simulink model "run_sim_paper_scenario"  (R2020a)
settings: Solver=ode4  StartTime=0.0  StopTime=30.0  FixedStep=0.01  RelTol=1e-3
values from neighbouring files (symbols this model uses):
  alfa_theta = 20    [init_sim_paper_scenario.m]
  alfa_theta_obs = 100    [init_sim_paper_scenario.m]
  beta1 = 1.2    [init_sim_paper_scenario.m]
  beta2 = 0.8    [init_sim_paper_scenario.m]
  beta_Phi_1 = pp0 * cal_frac_squ( 3, p_p0_plus_1, q_p0_plus_1 )                          * cal_frac_squ( eps_s_bar / pi, p_p0_min_2, q_p0_min_2 )                          / ( 2 * ( 2 * pp0 - 1 ) * tanh( gamma0 * ( eps_s_bar / pi ) / 2 ) )                          - ( cal_frac_squ( 3, p_p0_plus_1, q_p0_plus_1 ) * gamma0 / ( 4 * ( 2 * pp0 -1 ) ) )                          * cal_frac_squ( eps_s_bar / pi, p_p0_min_ ...(+136 chars)    [init_sim_paper_scenario.m]
  beta_Phi_2 = ( 1 - pp0 ) * cal_frac_squ( 3, p_p0_plus_1, q_p0_plus_1 )                          / ( 2 * ( 1 - 2 * pp0 ) * cal_frac_squ( eps_s_bar / pi, p_p0_0, q_p0_0 ) * tanh( gamma0 * ( eps_s_bar / pi ) / 2 ) )                          - ( cal_frac_squ( 3, p_p0_plus_1, q_p0_plus_1 ) * gamma0 / ( 4 * ( 1 - 2 * pp0 ) ) )                          * cal_frac_squ( eps_s_bar / pi, p_1_min_p0, q_1_min_p0 )          ...(+112 chars)    [init_sim_paper_scenario.m]
  c1_diff_sigma_bar_v = diag([25; 30; 20])    [init_sim_paper_scenario.m]
  c1_diff_sigma_bar_w = diag([12; 12; 12])    [init_sim_paper_scenario.m]
  c1_diff_ui = diag([25; 30; 20])    [init_sim_paper_scenario.m]
  c1v = diag([5.8; 6.5; 6.5])    [init_sim_paper_scenario.m]
  c2_diff_sigma_bar_v = diag([50; 50; 10])    [init_sim_paper_scenario.m]
  c2_diff_sigma_bar_w = diag([12; 12; 12])    [init_sim_paper_scenario.m]
  c2_diff_ui = diag([50; 50; 10])    [init_sim_paper_scenario.m]
  c2v = diag([5.8; 6.5; 6.5])    [init_sim_paper_scenario.m]
  c3_diff_sigma_bar_v = diag([15; 15; 10])    [init_sim_paper_scenario.m]
  c3_diff_sigma_bar_w = diag([15; 15; 15])    [init_sim_paper_scenario.m]
  c3_diff_ui = diag([15; 15; 10])    [init_sim_paper_scenario.m]
  c3v = diag([4.8; 6.4; 6.0])    [init_sim_paper_scenario.m]
  c_w_1 = diag( [20; 15; 15] )    [init_sim_paper_scenario.m]
  c_w_2 = diag( [20; 15; 15] )    [init_sim_paper_scenario.m]
  c_w_3 = diag( [2; 2; 2] )    [init_sim_paper_scenario.m]
  cS0 = diag( [4.5; 4.5; 4.5] )    [init_sim_paper_scenario.m]
  delta_p_i_0 = zeros(3, NF)    [init_sim_paper_scenario.m]
  delta_v_i_0 = zeros(3, NF)    [init_sim_paper_scenario.m]
  dp_aa_t = 0.2 * ones(3, 5) + ( 1.0 - 0.2 ) * rand(3, 5)    [init_sim_paper_scenario.m]
  dp_ff_t = [ 0.4 * ones(1, 5) + ( 1.0 - 0.4 ) * rand(1, 5);                      0.4 * ones(1, 5) + ( 1.0 - 0.4 ) * rand(1, 5);                      0.2 * ones(1, 5) + ( 0.6 - 0.2 ) * rand(1, 5) ]    [init_sim_paper_scenario.m]
  dp_phi_t = ( - pi / 2 ) * ones(3, 5) + ( pi / 2 - ( - pi / 2 ) ) * rand(3, 5)    [init_sim_paper_scenario.m]
  dw_aa_t = 0.2 * ones(3, 5) + ( 1.0 - 0.2 ) * rand(3, 5)    [init_sim_paper_scenario.m]
  dw_ff_t = [ 0.4 * ones(1, 5) + ( 1.0 - 0.4 ) * rand(1, 5);                      0.4 * ones(1, 5) + ( 1.0 - 0.4 ) * rand(1, 5);                      0.2 * ones(1, 5) + ( 0.6 - 0.2 ) * rand(1, 5) ]    [init_sim_paper_scenario.m]
  dw_phi_t = ( - pi / 2 ) * ones(3, 5) + ( pi / 2 - ( - pi / 2 ) ) * rand(3, 5)    [init_sim_paper_scenario.m]
  dwci_init = zeros(3,5)    [init_sim_paper_scenario.m]
  eps_s_bar_div_pi = eps_s_bar / pi    (= 0.03)    [init_sim_paper_scenario.m]
  etai_0 = zeros(3,5)    [init_sim_paper_scenario.m]
  gamma0 = 20    [init_sim_paper_scenario.m]
  h1w = diag([20.0; 20.0; 20.0])    [init_sim_paper_scenario.m]
  h2w = diag([30.0; 35.0; 35.0])    [init_sim_paper_scenario.m]
  h3w = diag([30.0; 25.0; 30.0])    [init_sim_paper_scenario.m]
  Ji = zeros(3,3,NF)    [init_sim_paper_scenario.m]
  k_J_0 = diag( [1; 1; 1] )    [init_sim_paper_scenario.m]
  kai_1_t = 0.02    [init_sim_paper_scenario.m]
  kai_3_t = 0.1    [init_sim_paper_scenario.m]
  kai_chi_1 = diag([6; 6; 6])    [init_sim_paper_scenario.m]
  kai_chi_2 = diag([6; 6; 6])    [init_sim_paper_scenario.m]
  kai_u_1 = diag([8; 8; 8])    [init_sim_paper_scenario.m]
  kai_u_2 = diag([8; 8; 8])    [init_sim_paper_scenario.m]
  ksii_0 = zeros(3,5)    [init_sim_paper_scenario.m]
  l1v = diag([20; 20; 20])    [init_sim_paper_scenario.m]
  l2v = diag([30; 30; 30])    [init_sim_paper_scenario.m]
  Lamd_diff_sigma_bar_v = 0.5    [init_sim_paper_scenario.m]
  Lamd_diff_sigma_bar_w = 0.8    [init_sim_paper_scenario.m]
  Lamd_diff_ui = 0.8    [init_sim_paper_scenario.m]
  mass_i = zeros(1,NF)    [init_sim_paper_scenario.m]
  Mii = diag([1;0;0;0;1])    [init_sim_paper_scenario.m]
  mu_c_theta = 100    [init_sim_paper_scenario.m]
  mu_d_w = 100    [init_sim_paper_scenario.m]
  pos0 = zeros(3, 1)    [init_sim_paper_scenario.m]
  pp0 = 8 / 11    (= 0.727272727273)    [init_sim_paper_scenario.m]    (also in plot_sim_paper_scenario.m = plot3( ksi0(1, kkt), ksi0(2, kkt), ksi0(3, kkt),            )
  PZ0 = P0(3)    [init_sim_paper_scenario.m]
  PZ1 = 10    [init_sim_paper_scenario.m]
  Qci_init = repmat([1;0;0;0],1,NF)    [init_sim_paper_scenario.m]
  R0 = 4    [init_sim_paper_scenario.m]
  R1 = 8    [init_sim_paper_scenario.m]
  Rci_init = zeros(3,3,NF)    [init_sim_paper_scenario.m]
  Ri_init = zeros(3,3,NF)    [init_sim_paper_scenario.m]
  Rx2 = 10    [init_sim_paper_scenario.m]
  Ry2 = 6    [init_sim_paper_scenario.m]
  Rz2 = 4    [init_sim_paper_scenario.m]
  T0 = 0    [init_sim_paper_scenario.m]
  T1 = tseq1    (= 10)    [init_sim_paper_scenario.m]
  T12 = tseq1 + tseq12    (= 20)    [init_sim_paper_scenario.m]
  T2 = tseq1 + tseq12 + tseq2    (= 30)    [init_sim_paper_scenario.m]
  theta0 = ( 2 / 5 ) * pi    (= 1.25663706144)    [init_sim_paper_scenario.m]
  thr_p_plus_1 = cal_frac_squ( 3, p_p0_plus_1, q_p0_plus_1 )    [init_sim_paper_scenario.m]
  ui_init = zeros(3,NF)    [init_sim_paper_scenario.m]
  vel0 = zeros(3, 1)    [init_sim_paper_scenario.m]
  wci_init = zeros(3,5)    [init_sim_paper_scenario.m]
  Wij = [0,0,1,0,0;              0,0,1,1,0;              1,0,0,0,1;              0,1,1,0,0;              0,0,1,0,0]    [init_sim_paper_scenario.m]
  X1 = 8    [init_sim_paper_scenario.m]
  X2 = 2    [init_sim_paper_scenario.m]
  X3 = 3    [init_sim_paper_scenario.m]
  Y1 = 10    [init_sim_paper_scenario.m]
  Y2 = 2    [init_sim_paper_scenario.m]
  Y3 = 4    [init_sim_paper_scenario.m]
  Z1 = 4    [init_sim_paper_scenario.m]
  Z2 = -6    [init_sim_paper_scenario.m]
  Z3 = 2    [init_sim_paper_scenario.m]
  zeta_diff_sigma_bar_v = 0.08    [init_sim_paper_scenario.m]
  zeta_diff_sigma_bar_w = 0.3    [init_sim_paper_scenario.m]
  zeta_diff_ui = 0.05    [init_sim_paper_scenario.m]
undefined symbols (not defined in the file or in its folder): cal_frac_squ, p_2_p0, p_alfav1, p_alfav2, p_alfaw1, p_alfaw2, p_beta1, p_beta2, p_beta_w_1, p_beta_w_2, p_dbeta1, p_dbeta2, p_gamma1_pos, p_gamma1_vel, p_gamma2_pos, p_gamma2_vel, p_p0_min_1, p_p0_plus_1, q_2_p0, q_alfav1, q_alfav2, q_alfaw1, q_alfaw2, q_beta1, q_beta2, q_beta_w_1, q_beta_w_2, q_dbeta1, q_dbeta2, q_gamma1_pos, q_gamma1_vel, q_gamma2_pos, q_gamma2_vel, q_p0_min_1, q_p0_plus_1, Qei_init, Qi_init, Rei_init, V_Phi_Rei_init, wei_init, wi_init
(part 9 of 10)

== matlab function run_sim_paper_scenario/cal taui agent 1 ==
  data: c_w_1 input; c_w_2 input; c_w_3 input; k_J_0 input; tau_1 output; Ji input; Si_vec input; dw_hat_vec input; Fi_S_vec input; theta_Si_beta_w_1_vec input; theta_Si_beta_w_2_vec input
function tau_1 = fcn(c_w_1, c_w_2, c_w_3, k_J_0, Ji, Si_vec, dw_hat_vec, ...
                                        Fi_S_vec, theta_Si_beta_w_1_vec, theta_Si_beta_w_2_vec)
%%%% applied torque control input for rotational subsystem
iiuav = 1;
tau_1 = -c_w_1 * theta_Si_beta_w_1_vec(:,iiuav) - c_w_2 * theta_Si_beta_w_2_vec(:,iiuav) - c_w_3 * Si_vec(:,iiuav) ...
                - dw_hat_vec(:,iiuav) - k_J_0 * inv( Ji(:,:,iiuav) ) * Fi_S_vec(:,iiuav);
end

== matlab function run_sim_paper_scenario/cal taui agent 2 ==
  data: c_w_1 input; c_w_2 input; c_w_3 input; k_J_0 input; tau_2 output; Ji input; Si_vec input; dw_hat_vec input; Fi_S_vec input; theta_Si_beta_w_1_vec input; theta_Si_beta_w_2_vec input
function tau_2 = fcn(c_w_1, c_w_2, c_w_3, k_J_0, Ji, Si_vec, dw_hat_vec, ...
                                        Fi_S_vec, theta_Si_beta_w_1_vec, theta_Si_beta_w_2_vec)
%%%% applied torque control input for rotational subsystem
iiuav = 2;
tau_2 = -c_w_1 * theta_Si_beta_w_1_vec(:,iiuav) - c_w_2 * theta_Si_beta_w_2_vec(:,iiuav) - c_w_3 * Si_vec(:,iiuav) ...
                - dw_hat_vec(:,iiuav) - k_J_0 * inv( Ji(:,:,iiuav) ) * Fi_S_vec(:,iiuav);
end

== matlab function run_sim_paper_scenario/cal taui agent 3 ==
  data: c_w_1 input; c_w_2 input; c_w_3 input; k_J_0 input; tau_3 output; Ji input; Si_vec input; dw_hat_vec input; Fi_S_vec input; theta_Si_beta_w_1_vec input; theta_Si_beta_w_2_vec input
function tau_3 = fcn(c_w_1, c_w_2, c_w_3, k_J_0, Ji, Si_vec, dw_hat_vec, ...
                                        Fi_S_vec, theta_Si_beta_w_1_vec, theta_Si_beta_w_2_vec)
%%%% applied torque control input for rotational subsystem
iiuav = 3;
tau_3 = -c_w_1 * theta_Si_beta_w_1_vec(:,iiuav) - c_w_2 * theta_Si_beta_w_2_vec(:,iiuav) - c_w_3 * Si_vec(:,iiuav) ...
                - dw_hat_vec(:,iiuav) - k_J_0 * inv( Ji(:,:,iiuav) ) * Fi_S_vec(:,iiuav);
end

== matlab function run_sim_paper_scenario/cal taui agent 4 ==
  data: c_w_1 input; c_w_2 input; c_w_3 input; k_J_0 input; tau_4 output; Ji input; Si_vec input; dw_hat_vec input; Fi_S_vec input; theta_Si_beta_w_1_vec input; theta_Si_beta_w_2_vec input
function tau_4 = fcn(c_w_1, c_w_2, c_w_3, k_J_0, Ji, Si_vec, dw_hat_vec, ...
                                        Fi_S_vec, theta_Si_beta_w_1_vec, theta_Si_beta_w_2_vec)
%%%% applied torque control input for rotational subsystem
iiuav = 4;
tau_4 = -c_w_1 * theta_Si_beta_w_1_vec(:,iiuav) - c_w_2 * theta_Si_beta_w_2_vec(:,iiuav) - c_w_3 * Si_vec(:,iiuav) ...
                - dw_hat_vec(:,iiuav) - k_J_0 * inv( Ji(:,:,iiuav) ) * Fi_S_vec(:,iiuav);
end

== matlab function run_sim_paper_scenario/cal taui agent 5 ==
  data: c_w_1 input; c_w_2 input; c_w_3 input; k_J_0 input; tau_5 output; Ji input; Si_vec input; dw_hat_vec input; Fi_S_vec input; theta_Si_beta_w_1_vec input; theta_Si_beta_w_2_vec input
function tau_5 = fcn(c_w_1, c_w_2, c_w_3, k_J_0, Ji, Si_vec, dw_hat_vec, ...
                                        Fi_S_vec, theta_Si_beta_w_1_vec, theta_Si_beta_w_2_vec)
%%%% applied torque control input for rotational subsystem
iiuav = 5;
tau_5 = -c_w_1 * theta_Si_beta_w_1_vec(:,iiuav) - c_w_2 * theta_Si_beta_w_2_vec(:,iiuav) - c_w_3 * Si_vec(:,iiuav) ...
                - dw_hat_vec(:,iiuav) - k_J_0 * inv( Ji(:,:,iiuav) ) * Fi_S_vec(:,iiuav);
end

== matlab function run_sim_paper_scenario/cal theta_Si_beta_w agent 1 ==
  data: mu_c_theta input; Si_squ_beta_w_1_vec input; theta_Si_beta_w_1_node_1 output; Si_squ_beta_w_2_vec input; Si_vec input; theta_Si_beta_w_2_node_1 output
function [theta_Si_beta_w_1_node_1, theta_Si_beta_w_2_node_1] = fcn(mu_c_theta, Si_squ_beta_w_1_vec, Si_squ_beta_w_2_vec, Si_vec)
iiuav = 1;
theta_Si_beta_w_1_node_1 = Si_squ_beta_w_1_vec(:, iiuav) .* ( -1 + 2 ./ ( 1 + exp( -mu_c_theta .* Si_vec(:,iiuav) ) ) );
theta_Si_beta_w_2_node_1 = Si_squ_beta_w_2_vec(:, iiuav) .* ( -1 + 2 ./ ( 1 + exp( -mu_c_theta .* Si_vec(:,iiuav) ) ) );

== matlab function run_sim_paper_scenario/cal theta_Si_beta_w agent 2 ==
  data: mu_c_theta input; Si_squ_beta_w_1_vec input; theta_Si_beta_w_1_node_2 output; Si_squ_beta_w_2_vec input; Si_vec input; theta_Si_beta_w_2_node_2 output
function [theta_Si_beta_w_1_node_2, theta_Si_beta_w_2_node_2] = fcn(mu_c_theta, Si_squ_beta_w_1_vec, Si_squ_beta_w_2_vec, Si_vec)
iiuav = 2;
theta_Si_beta_w_1_node_2 = Si_squ_beta_w_1_vec(:, iiuav) .* ( -1 + 2 ./ ( 1 + exp( -mu_c_theta .* Si_vec(:,iiuav) ) ) );
theta_Si_beta_w_2_node_2 = Si_squ_beta_w_2_vec(:, iiuav) .* ( -1 + 2 ./ ( 1 + exp( -mu_c_theta .* Si_vec(:,iiuav) ) ) );

== matlab function run_sim_paper_scenario/combine follower eta ksi ==
  data: ksi_track_err_vec output; ksi_track_err_1 input; ksi_track_err_2 input; ksi_track_err_3 input; ksi_track_err_4 input; ksi_track_err_5 input; eta_track_err_vec output; eta_track_err_1 input; eta_track_err_2 input; eta_track_err_3 input; eta_track_err_4 input; eta_track_err_5 input
function [ksi_track_err_vec, eta_track_err_vec]  = fcn(ksi_track_err_1, ksi_track_err_2, ksi_track_err_3, ksi_track_err_4, ksi_track_err_5, ...
                                                                                    eta_track_err_1, eta_track_err_2, eta_track_err_3, eta_track_err_4, eta_track_err_5)
ksi_track_err_vec = [ksi_track_err_1(:), ksi_track_err_2(:), ksi_track_err_3(:), ksi_track_err_4(:), ksi_track_err_5(:)];
eta_track_err_vec = [eta_track_err_1(:), eta_track_err_2(:), eta_track_err_3(:), eta_track_err_4(:), eta_track_err_5(:)];

== matlab function run_sim_paper_scenario/cal theta_Si_beta_w agent 3 ==
  data: mu_c_theta input; Si_squ_beta_w_1_vec input; theta_Si_beta_w_1_node_3 output; Si_squ_beta_w_2_vec input; Si_vec input; theta_Si_beta_w_2_node_3 output
function [theta_Si_beta_w_1_node_3, theta_Si_beta_w_2_node_3] = fcn(mu_c_theta, Si_squ_beta_w_1_vec, Si_squ_beta_w_2_vec, Si_vec)
iiuav = 3;
theta_Si_beta_w_1_node_3 = Si_squ_beta_w_1_vec(:, iiuav) .* ( -1 + 2 ./ ( 1 + exp( -mu_c_theta .* Si_vec(:,iiuav) ) ) );
theta_Si_beta_w_2_node_3 = Si_squ_beta_w_2_vec(:, iiuav) .* ( -1 + 2 ./ ( 1 + exp( -mu_c_theta .* Si_vec(:,iiuav) ) ) );

== matlab function run_sim_paper_scenario/cal theta_Si_beta_w agent 4 ==
  data: mu_c_theta input; Si_squ_beta_w_1_vec input; theta_Si_beta_w_1_node_4 output; Si_squ_beta_w_2_vec input; Si_vec input; theta_Si_beta_w_2_node_4 output
function [theta_Si_beta_w_1_node_4, theta_Si_beta_w_2_node_4] = fcn(mu_c_theta, Si_squ_beta_w_1_vec, Si_squ_beta_w_2_vec, Si_vec)
iiuav = 4;
theta_Si_beta_w_1_node_4 = Si_squ_beta_w_1_vec(:, iiuav) .* ( -1 + 2 ./ ( 1 + exp( -mu_c_theta .* Si_vec(:,iiuav) ) ) );
theta_Si_beta_w_2_node_4 = Si_squ_beta_w_2_vec(:, iiuav) .* ( -1 + 2 ./ ( 1 + exp( -mu_c_theta .* Si_vec(:,iiuav) ) ) );

== matlab function run_sim_paper_scenario/cal theta_Si_beta_w agent 5 ==
  data: mu_c_theta input; Si_squ_beta_w_1_vec input; theta_Si_beta_w_1_node_5 output; Si_squ_beta_w_2_vec input; Si_vec input; theta_Si_beta_w_2_node_5 output
function [theta_Si_beta_w_1_node_5, theta_Si_beta_w_2_node_5] = fcn(mu_c_theta, Si_squ_beta_w_1_vec, Si_squ_beta_w_2_vec, Si_vec)
iiuav = 5;
theta_Si_beta_w_1_node_5 = Si_squ_beta_w_1_vec(:, iiuav) .* ( -1 + 2 ./ ( 1 + exp( -mu_c_theta .* Si_vec(:,iiuav) ) ) );
theta_Si_beta_w_2_node_5 = Si_squ_beta_w_2_vec(:, iiuav) .* ( -1 + 2 ./ ( 1 + exp( -mu_c_theta .* Si_vec(:,iiuav) ) ) );

== matlab function run_sim_paper_scenario/cal theta_sigma_bar_w_tilt agent 1 ==
  data: alfa_theta_obs_w input; sigma_bar_w_tilt_squ_1_1 input; theta_sigma_bar_w_tilt_1_1 output; sigma_bar_w_tilt_squ_2_1 input; sigma_bar_w_tilt_vec input; theta_sigma_bar_w_tilt_2_1 output
function [theta_sigma_bar_w_tilt_1_1, theta_sigma_bar_w_tilt_2_1] = fcn(alfa_theta_obs_w, sigma_bar_w_tilt_squ_1_1, sigma_bar_w_tilt_squ_2_1, sigma_bar_w_tilt_vec)
iiuav = 1;
theta_sigma_bar_w_tilt_1_1 = sigma_bar_w_tilt_squ_1_1(:) .* ( -1 + 2 ./ ( 1 + exp( -alfa_theta_obs_w .* sigma_bar_w_tilt_vec(:,iiuav) ) ) );
theta_sigma_bar_w_tilt_2_1 = sigma_bar_w_tilt_squ_2_1(:) .* ( -1 + 2 ./ ( 1 + exp( -alfa_theta_obs_w .* sigma_bar_w_tilt_vec(:,iiuav) ) ) );

== matlab function run_sim_paper_scenario/cal theta_sigma_bar_w_tilt agent 2 ==
  data: alfa_theta_obs_w input; sigma_bar_w_tilt_squ_1_2 input; theta_sigma_bar_w_tilt_1_2 output; sigma_bar_w_tilt_squ_2_2 input; sigma_bar_w_tilt_vec input; theta_sigma_bar_w_tilt_2_2 output
function [theta_sigma_bar_w_tilt_1_2, theta_sigma_bar_w_tilt_2_2] = fcn(alfa_theta_obs_w, sigma_bar_w_tilt_squ_1_2, sigma_bar_w_tilt_squ_2_2, sigma_bar_w_tilt_vec)
iiuav = 2;
theta_sigma_bar_w_tilt_1_2 = sigma_bar_w_tilt_squ_1_2(:) .* ( -1 + 2 ./ ( 1 + exp( -alfa_theta_obs_w .* sigma_bar_w_tilt_vec(:,iiuav) ) ) );
theta_sigma_bar_w_tilt_2_2 = sigma_bar_w_tilt_squ_2_2(:) .* ( -1 + 2 ./ ( 1 + exp( -alfa_theta_obs_w .* sigma_bar_w_tilt_vec(:,iiuav) ) ) );

== matlab function run_sim_paper_scenario/cal theta_sigma_bar_w_tilt agent 3 ==
  data: alfa_theta_obs_w input; sigma_bar_w_tilt_squ_1_3 input; theta_sigma_bar_w_tilt_1_3 output; sigma_bar_w_tilt_squ_2_3 input; sigma_bar_w_tilt_vec input; theta_sigma_bar_w_tilt_2_3 output
function [theta_sigma_bar_w_tilt_1_3, theta_sigma_bar_w_tilt_2_3] = fcn(alfa_theta_obs_w, sigma_bar_w_tilt_squ_1_3, sigma_bar_w_tilt_squ_2_3, sigma_bar_w_tilt_vec)
iiuav = 3;
theta_sigma_bar_w_tilt_1_3 = sigma_bar_w_tilt_squ_1_3(:) .* ( -1 + 2 ./ ( 1 + exp( -alfa_theta_obs_w .* sigma_bar_w_tilt_vec(:,iiuav) ) ) );
theta_sigma_bar_w_tilt_2_3 = sigma_bar_w_tilt_squ_2_3(:) .* ( -1 + 2 ./ ( 1 + exp( -alfa_theta_obs_w .* sigma_bar_w_tilt_vec(:,iiuav) ) ) );

== matlab function run_sim_paper_scenario/cal theta_sigma_bar_w_tilt agent 4 ==
  data: alfa_theta_obs_w input; sigma_bar_w_tilt_squ_1_4 input; theta_sigma_bar_w_tilt_1_4 output; sigma_bar_w_tilt_squ_2_4 input; sigma_bar_w_tilt_vec input; theta_sigma_bar_w_tilt_2_4 output
function [theta_sigma_bar_w_tilt_1_4, theta_sigma_bar_w_tilt_2_4] = fcn(alfa_theta_obs_w, sigma_bar_w_tilt_squ_1_4, sigma_bar_w_tilt_squ_2_4, sigma_bar_w_tilt_vec)
iiuav = 4;
theta_sigma_bar_w_tilt_1_4 = sigma_bar_w_tilt_squ_1_4(:) .* ( -1 + 2 ./ ( 1 + exp( -alfa_theta_obs_w .* sigma_bar_w_tilt_vec(:,iiuav) ) ) );
theta_sigma_bar_w_tilt_2_4 = sigma_bar_w_tilt_squ_2_4(:) .* ( -1 + 2 ./ ( 1 + exp( -alfa_theta_obs_w .* sigma_bar_w_tilt_vec(:,iiuav) ) ) );

== matlab function run_sim_paper_scenario/cal theta_sigma_bar_w_tilt agent 5 ==
  data: alfa_theta_obs_w input; sigma_bar_w_tilt_squ_1_5 input; theta_sigma_bar_w_tilt_1_5 output; sigma_bar_w_tilt_squ_2_5 input; sigma_bar_w_tilt_vec input; theta_sigma_bar_w_tilt_2_5 output
function [theta_sigma_bar_w_tilt_1_5, theta_sigma_bar_w_tilt_2_5] = fcn(alfa_theta_obs_w, sigma_bar_w_tilt_squ_1_5, sigma_bar_w_tilt_squ_2_5, sigma_bar_w_tilt_vec)
iiuav = 5;
theta_sigma_bar_w_tilt_1_5 = sigma_bar_w_tilt_squ_1_5(:) .* ( -1 + 2 ./ ( 1 + exp( -alfa_theta_obs_w .* sigma_bar_w_tilt_vec(:,iiuav) ) ) );
theta_sigma_bar_w_tilt_2_5 = sigma_bar_w_tilt_squ_2_5(:) .* ( -1 + 2 ./ ( 1 + exp( -alfa_theta_obs_w .* sigma_bar_w_tilt_vec(:,iiuav) ) ) );

== matlab function run_sim_paper_scenario/cal wci dwci agent 1 ==
  data: ui_vec input; wci output; duihat_vec input; d2uihat_vec input; Rci_mat input; dwci output
function [wci, dwci] = fcn(ui_vec, duihat_vec, d2uihat_vec, Rci_mat)
%%%% Angular Velocity Command and its derivative

iiuav = 1;
ui = ui_vec(:,iiuav);
duihat = duihat_vec(:,iiuav);
d2uihat = d2uihat_vec(:,iiuav);
Rci = Rci_mat(:,:,iiuav);

ee1 = [1;0;0];
ee2 = [0;1;0];
ee3 = [0;0;1];
RciE3 = ui / norm(ui,2);
PiMat = eye(3,3) - ee3*(ee3');
dRciE3 = (1 / norm(ui,2))*Rci*PiMat*(Rci')*duihat;
Themat = [-RciE3(2)/(1+RciE3(3)),         -RciE3(1)/(1+RciE3(3)),       (RciE3(1)*RciE3(2))/((1+RciE3(3))^2); ...
                   2*RciE3(1)/(1+RciE3(3)),                0,                               1 - (RciE3(1)^2)/((1+RciE3(3))^2); ...
                               0                                       -1                                                        0                                   ];
wcxe3 = (1 / norm(ui,2))*PiMat*(Rci')*duihat;
wcxe2 = (1 / norm(ui,2))*(Rci')*Themat*Rci*PiMat*(Rci')*duihat;
wci = [-wcxe3(2); wcxe3(1); -wcxe2(1)];

TempMat1 = [0,                           -1/(1+RciE3(3)),                   (RciE3(2))/((1+RciE3(3))^2); ...
                       2/(1+RciE3(3)),                0,                               (-2*RciE3(1))/((1+RciE3(3))^2); ...
                       0,                                     0,                                                   0                             ];
TempMat2 = [-1/(1+RciE3(3)),              0,                               (RciE3(1))/((1+RciE3(3))^2); ...
                       0,                                     0,                                                   0                      ; ...
                       0,                                     0,                                                   0                             ];
TempMat3 = [(RciE3(2))/((1+RciE3(3))^2),                 (RciE3(1))/((1+RciE3(3))^2),       (-2*RciE3(1)*RciE3(2))/((1+RciE3(3))^3); ...
                       (-2*RciE3(1))/((1+RciE3(3))^2),                             0,                               (2*(RciE3(1)^2))/((1+RciE3(3))^3); ...
                        0,                                                                          0,                                                   0                             ];
dTheMat = TempMat1*dRciE3*(ee1') + TempMat2*dRciE3*(ee2') + TempMat3*dRciE3*(ee3');
wcix = cal_askew_mat(wci);
dRciT = -wcix*(Rci');
dwcxe3 = (1 / norm(ui,2))*PiMat*(dRciT*duihat+(Rci')*(d2uihat-(((ui')*duihat)/(norm(ui,2)^2))*duihat));
dwcxe2 = (1 / norm(ui,2))*((dRciT*Themat+(Rci')*dTheMat) ...
                *(Rci*PiMat*(Rci'))*duihat + (Rci')*Themat*(Rci*PiMat*(Rci'))*(d2uihat-(((ui')*duihat)/(norm(ui,2)^2))*duihat));
dwci = [-dwcxe3(2);  dwcxe3(1);  -dwcxe2(1)];

== matlab function run_sim_paper_scenario/cal wci dwci agent 2 ==
  data: ui_vec input; wci output; duihat_vec input; d2uihat_vec input; Rci_mat input; dwci output
function [wci, dwci] = fcn(ui_vec, duihat_vec, d2uihat_vec, Rci_mat)
%%%% Angular Velocity Command and its derivative

iiuav = 2;
ui = ui_vec(:,iiuav);
duihat = duihat_vec(:,iiuav);
d2uihat = d2uihat_vec(:,iiuav);
Rci = Rci_mat(:,:,iiuav);

ee1 = [1;0;0];
ee2 = [0;1;0];
ee3 = [0;0;1];
RciE3 = ui / norm(ui,2);
PiMat = eye(3,3) - ee3*(ee3');
dRciE3 = (1 / norm(ui,2))*Rci*PiMat*(Rci')*duihat;
Themat = [-RciE3(2)/(1+RciE3(3)),         -RciE3(1)/(1+RciE3(3)),       (RciE3(1)*RciE3(2))/((1+RciE3(3))^2); ...
                   2*RciE3(1)/(1+RciE3(3)),                0,                               1 - (RciE3(1)^2)/((1+RciE3(3))^2); ...
                               0                                       -1                                                        0                                   ];
wcxe3 = (1 / norm(ui,2))*PiMat*(Rci')*duihat;
wcxe2 = (1 / norm(ui,2))*(Rci')*Themat*Rci*PiMat*(Rci')*duihat;
wci = [-wcxe3(2); wcxe3(1); -wcxe2(1)];

TempMat1 = [0,                           -1/(1+RciE3(3)),                   (RciE3(2))/((1+RciE3(3))^2); ...
                       2/(1+RciE3(3)),                0,                               (-2*RciE3(1))/((1+RciE3(3))^2); ...
                       0,                                     0,                                                   0                             ];
TempMat2 = [-1/(1+RciE3(3)),              0,                               (RciE3(1))/((1+RciE3(3))^2); ...
                       0,                                     0,                                                   0                      ; ...
                       0,                                     0,                                                   0                             ];
TempMat3 = [(RciE3(2))/((1+RciE3(3))^2),                 (RciE3(1))/((1+RciE3(3))^2),       (-2*RciE3(1)*RciE3(2))/((1+RciE3(3))^3); ...
                       (-2*RciE3(1))/((1+RciE3(3))^2),                             0,                               (2*(RciE3(1)^2))/((1+RciE3(3))^3); ...
                        0,                                                                          0,                                                   0                             ];
dTheMat = TempMat1*dRciE3*(ee1') + TempMat2*dRciE3*(ee2') + TempMat3*dRciE3*(ee3');
wcix = cal_askew_mat(wci);
dRciT = -wcix*(Rci');
dwcxe3 = (1 / norm(ui,2))*PiMat*(dRciT*duihat+(Rci')*(d2uihat-(((ui')*duihat)/(norm(ui,2)^2))*duihat));
dwcxe2 = (1 / norm(ui,2))*((dRciT*Themat+(Rci')*dTheMat) ...
                *(Rci*PiMat*(Rci'))*duihat + (Rci')*Themat*(Rci*PiMat*(Rci'))*(d2uihat-(((ui')*duihat)/(norm(ui,2)^2))*duihat));
dwci = [-dwcxe3(2);  dwcxe3(1);  -dwcxe2(1)];

== matlab function run_sim_paper_scenario/cal wci dwci agent 3 ==
  data: ui_vec input; wci output; duihat_vec input; d2uihat_vec input; Rci_mat input; dwci output
function [wci, dwci] = fcn(ui_vec, duihat_vec, d2uihat_vec, Rci_mat)
%%%% Angular Velocity Command and its derivative

iiuav = 3;
ui = ui_vec(:,iiuav);
duihat = duihat_vec(:,iiuav);
d2uihat = d2uihat_vec(:,iiuav);
Rci = Rci_mat(:,:,iiuav);

ee1 = [1;0;0];
ee2 = [0;1;0];
ee3 = [0;0;1];
RciE3 = ui / norm(ui,2);
PiMat = eye(3,3) - ee3*(ee3');
dRciE3 = (1 / norm(ui,2))*Rci*PiMat*(Rci')*duihat;
Themat = [-RciE3(2)/(1+RciE3(3)),         -RciE3(1)/(1+RciE3(3)),       (RciE3(1)*RciE3(2))/((1+RciE3(3))^2); ...
                   2*RciE3(1)/(1+RciE3(3)),                0,                               1 - (RciE3(1)^2)/((1+RciE3(3))^2); ...
                               0                                       -1                                                        0                                   ];
wcxe3 = (1 / norm(ui,2))*PiMat*(Rci')*duihat;
wcxe2 = (1 / norm(ui,2))*(Rci')*Themat*Rci*PiMat*(Rci')*duihat;
wci = [-wcxe3(2); wcxe3(1); -wcxe2(1)];

TempMat1 = [0,                           -1/(1+RciE3(3)),                   (RciE3(2))/((1+RciE3(3))^2); ...
                       2/(1+RciE3(3)),                0,                               (-2*RciE3(1))/((1+RciE3(3))^2); ...
                       0,                                     0,                                                   0                             ];
TempMat2 = [-1/(1+RciE3(3)),              0,                               (RciE3(1))/((1+RciE3(3))^2); ...
                       0,                                     0,                                                   0                      ; ...
                       0,                                     0,                                                   0                             ];
TempMat3 = [(RciE3(2))/((1+RciE3(3))^2),                 (RciE3(1))/((1+RciE3(3))^2),       (-2*RciE3(1)*RciE3(2))/((1+RciE3(3))^3); ...
                       (-2*RciE3(1))/((1+RciE3(3))^2),                             0,                               (2*(RciE3(1)^2))/((1+RciE3(3))^3); ...
                        0,                                                                          0,                                                   0                             ];
dTheMat = TempMat1*dRciE3*(ee1') + TempMat2*dRciE3*(ee2') + TempMat3*dRciE3*(ee3');
wcix = cal_askew_mat(wci);
dRciT = -wcix*(Rci');
dwcxe3 = (1 / norm(ui,2))*PiMat*(dRciT*duihat+(Rci')*(d2uihat-(((ui')*duihat)/(norm(ui,2)^2))*duihat));
dwcxe2 = (1 / norm(ui,2))*((dRciT*Themat+(Rci')*dTheMat) ...
                *(Rci*PiMat*(Rci'))*duihat + (Rci')*Themat*(Rci*PiMat*(Rci'))*(d2uihat-(((ui')*duihat)/(norm(ui,2)^2))*duihat));
dwci = [-dwcxe3(2);  dwcxe3(1);  -dwcxe2(1)];

== matlab function run_sim_paper_scenario/cal wci dwci agent 4 ==
  data: ui_vec input; wci output; duihat_vec input; d2uihat_vec input; Rci_mat input; dwci output
function [wci, dwci] = fcn(ui_vec, duihat_vec, d2uihat_vec, Rci_mat)
%%%% Angular Velocity Command and its derivative

iiuav = 4;
ui = ui_vec(:,iiuav);
duihat = duihat_vec(:,iiuav);
d2uihat = d2uihat_vec(:,iiuav);
Rci = Rci_mat(:,:,iiuav);

ee1 = [1;0;0];
ee2 = [0;1;0];
ee3 = [0;0;1];
RciE3 = ui / norm(ui,2);
PiMat = eye(3,3) - ee3*(ee3');
dRciE3 = (1 / norm(ui,2))*Rci*PiMat*(Rci')*duihat;
Themat = [-RciE3(2)/(1+RciE3(3)),         -RciE3(1)/(1+RciE3(3)),       (RciE3(1)*RciE3(2))/((1+RciE3(3))^2); ...
                   2*RciE3(1)/(1+RciE3(3)),                0,                               1 - (RciE3(1)^2)/((1+RciE3(3))^2); ...
                               0                                       -1                                                        0                                   ];
wcxe3 = (1 / norm(ui,2))*PiMat*(Rci')*duihat;
wcxe2 = (1 / norm(ui,2))*(Rci')*Themat*Rci*PiMat*(Rci')*duihat;
wci = [-wcxe3(2); wcxe3(1); -wcxe2(1)];

TempMat1 = [0,                           -1/(1+RciE3(3)),                   (RciE3(2))/((1+RciE3(3))^2); ...
                       2/(1+RciE3(3)),                0,                               (-2*RciE3(1))/((1+RciE3(3))^2); ...
                       0,                                     0,                                                   0                             ];
TempMat2 = [-1/(1+RciE3(3)),              0,                               (RciE3(1))/((1+RciE3(3))^2); ...
                       0,                                     0,                                                   0                      ; ...
                       0,                                     0,                                                   0                             ];
TempMat3 = [(RciE3(2))/((1+RciE3(3))^2),                 (RciE3(1))/((1+RciE3(3))^2),       (-2*RciE3(1)*RciE3(2))/((1+RciE3(3))^3); ...
                       (-2*RciE3(1))/((1+RciE3(3))^2),                             0,                               (2*(RciE3(1)^2))/((1+RciE3(3))^3); ...
                        0,                                                                          0,                                                   0                             ];
dTheMat = TempMat1*dRciE3*(ee1') + TempMat2*dRciE3*(ee2') + TempMat3*dRciE3*(ee3');
wcix = cal_askew_mat(wci);
dRciT = -wcix*(Rci');
dwcxe3 = (1 / norm(ui,2))*PiMat*(dRciT*duihat+(Rci')*(d2uihat-(((ui')*duihat)/(norm(ui,2)^2))*duihat));
dwcxe2 = (1 / norm(ui,2))*((dRciT*Themat+(Rci')*dTheMat) ...
                *(Rci*PiMat*(Rci'))*duihat + (Rci')*Themat*(Rci*PiMat*(Rci'))*(d2uihat-(((ui')*duihat)/(norm(ui,2)^2))*duihat));
dwci = [-dwcxe3(2);  dwcxe3(1);  -dwcxe2(1)];

== matlab function run_sim_paper_scenario/cal wci dwci agent 5 ==
  data: ui_vec input; wci output; duihat_vec input; d2uihat_vec input; Rci_mat input; dwci output
function [wci, dwci] = fcn(ui_vec, duihat_vec, d2uihat_vec, Rci_mat)
%%%% Angular Velocity Command and its derivative

iiuav = 5;
ui = ui_vec(:,iiuav);
duihat = duihat_vec(:,iiuav);
d2uihat = d2uihat_vec(:,iiuav);
Rci = Rci_mat(:,:,iiuav);

ee1 = [1;0;0];
ee2 = [0;1;0];
ee3 = [0;0;1];
RciE3 = ui / norm(ui,2);
PiMat = eye(3,3) - ee3*(ee3');
dRciE3 = (1 / norm(ui,2))*Rci*PiMat*(Rci')*duihat;
Themat = [-RciE3(2)/(1+RciE3(3)),         -RciE3(1)/(1+RciE3(3)),       (RciE3(1)*RciE3(2))/((1+RciE3(3))^2); ...
                   2*RciE3(1)/(1+RciE3(3)),                0,                               1 - (RciE3(1)^2)/((1+RciE3(3))^2); ...
                               0                                       -1                                                        0                                   ];
wcxe3 = (1 / norm(ui,2))*PiMat*(Rci')*duihat;
wcxe2 = (1 / norm(ui,2))*(Rci')*Themat*Rci*PiMat*(Rci')*duihat;
wci = [-wcxe3(2); wcxe3(1); -wcxe2(1)];

TempMat1 = [0,                           -1/(1+RciE3(3)),                   (RciE3(2))/((1+RciE3(3))^2); ...
                       2/(1+RciE3(3)),                0,                               (-2*RciE3(1))/((1+RciE3(3))^2); ...
                       0,                                     0,                                                   0                             ];
TempMat2 = [-1/(1+RciE3(3)),              0,                               (RciE3(1))/((1+RciE3(3))^2); ...
                       0,                                     0,                                                   0                      ; ...
                       0,                                     0,                                                   0                             ];
TempMat3 = [(RciE3(2))/((1+RciE3(3))^2),                 (RciE3(1))/((1+RciE3(3))^2),       (-2*RciE3(1)*RciE3(2))/((1+RciE3(3))^3); ...
                       (-2*RciE3(1))/((1+RciE3(3))^2),                             0,                               (2*(RciE3(1)^2))/((1+RciE3(3))^3); ...
                        0,                                                                          0,                                                   0                             ];
dTheMat = TempMat1*dRciE3*(ee1') + TempMat2*dRciE3*(ee2') + TempMat3*dRciE3*(ee3');
wcix = cal_askew_mat(wci);
dRciT = -wcix*(Rci');
dwcxe3 = (1 / norm(ui,2))*PiMat*(dRciT*duihat+(Rci')*(d2uihat-(((ui')*duihat)/(norm(ui,2)^2))*duihat));
dwcxe2 = (1 / norm(ui,2))*((dRciT*Themat+(Rci')*dTheMat) ...
                *(Rci*PiMat*(Rci'))*duihat + (Rci')*Themat*(Rci*PiMat*(Rci'))*(d2uihat-(((ui')*duihat)/(norm(ui,2)^2))*duihat));
dwci = [-dwcxe3(2);  dwcxe3(1);  -dwcxe2(1)];

== matlab function run_sim_paper_scenario/cal wei agent 1 ==
  data: wi_vec input; wei_1 output; Rei_vec input; wci_vec input
function wei_1 = fcn(wi_vec, Rei_vec, wci_vec)
%%%% update angular velocity error
iiuav = 1;
wei_1 = wi_vec(:,iiuav) - (Rei_vec(:,:,iiuav)') * wci_vec(:,iiuav);

end

== matlab function run_sim_paper_scenario/cal wei agent 2 ==
  data: wi_vec input; wei_2 output; Rei_vec input; wci_vec input
function wei_2 = fcn(wi_vec, Rei_vec, wci_vec)
%%%% update angular velocity error
iiuav = 2;
wei_2 = wi_vec(:,iiuav) - (Rei_vec(:,:,iiuav)') * wci_vec(:,iiuav);

end

== matlab function run_sim_paper_scenario/cal wei agent 3 ==
  data: wi_vec input; wei_3 output; Rei_vec input; wci_vec input
function wei_3 = fcn(wi_vec, Rei_vec, wci_vec)
%%%% update angular velocity error
iiuav = 3;
wei_3 = wi_vec(:,iiuav) - (Rei_vec(:,:,iiuav)') * wci_vec(:,iiuav);

end

== matlab function run_sim_paper_scenario/cal abs 10 ==
  data: x input; y output
function y = fcn(x)
y = abs(x(:));

== matlab function run_sim_paper_scenario/cal wei agent 4 ==
  data: wi_vec input; wei_4 output; Rei_vec input; wci_vec input
function wei_4 = fcn(wi_vec, Rei_vec, wci_vec)
%%%% update angular velocity error
iiuav = 4;
wei_4 = wi_vec(:,iiuav) - (Rei_vec(:,:,iiuav)') * wci_vec(:,iiuav);

end

== matlab function run_sim_paper_scenario/cal wei agent 5 ==
  data: wi_vec input; wei_5 output; Rei_vec input; wci_vec input
function wei_5 = fcn(wi_vec, Rei_vec, wci_vec)
%%%% update angular velocity error
iiuav = 5;
wei_5 = wi_vec(:,iiuav) - (Rei_vec(:,:,iiuav)') * wci_vec(:,iiuav);

end

== matlab function run_sim_paper_scenario/choose ksi_est_err 41 ==
  data: x input; y output
function y = fcn(x)
iiuav = 1;
y = x(:,iiuav);

== matlab function run_sim_paper_scenario/choose ksi_est_err 42 ==
  data: x input; y output
function y = fcn(x)
iiuav = 5;
y = x(:,iiuav);

== matlab function run_sim_paper_scenario/choose ksi_est_err 43 ==
  data: x input; y output
function y = fcn(x)
iiuav = 1;
y = x(:,iiuav);

== matlab function run_sim_paper_scenario/choose ksi_est_err 44 ==
  data: x input; y output
function y = fcn(x)
iiuav = 1;
y = x(:,iiuav);

== matlab function run_sim_paper_scenario/choose ksi_est_err 45 ==
  data: x input; y output
function y = fcn(x)
iiuav = 2;
y = x(:,iiuav);

== matlab function run_sim_paper_scenario/choose ksi_est_err 46 ==
  data: x input; y output
function y = fcn(x)
iiuav = 2;
y = x(:,iiuav);

== matlab function run_sim_paper_scenario/choose ksi_est_err 47 ==
  data: x input; y output
function y = fcn(x)
iiuav = 3;
y = x(:,iiuav);

== matlab function run_sim_paper_scenario/choose ksi_est_err 48 ==
  data: x input; y output
function y = fcn(x)
iiuav = 3;
y = x(:,iiuav);

== matlab function run_sim_paper_scenario/cal abs 9 ==
  data: x input; y output
function y = fcn(x)
y = abs(x(:));

== matlab function run_sim_paper_scenario/choose ksi_est_err 49 ==
  data: x input; y output
function y = fcn(x)
iiuav = 4;
y = x(:,iiuav);

== matlab function run_sim_paper_scenario/choose ksi_est_err 50 ==
  data: x input; y output
function y = fcn(x)
iiuav = 4;
y = x(:,iiuav);

== matlab function run_sim_paper_scenario/choose ksi_est_err 51 ==
  data: x input; y output
function y = fcn(x)
iiuav = 5;
y = x(:,iiuav);

== matlab function run_sim_paper_scenario/choose ksi_est_err 52 ==
  data: x input; y output
function y = fcn(x)
iiuav = 1;
y = x(:,iiuav);

== matlab function run_sim_paper_scenario/choose ksi_est_err 53 ==
  data: x input; y output
function y = fcn(x)
iiuav = 5;
y = x(:,iiuav);

== matlab function run_sim_paper_scenario/choose ksi_est_err 54 ==
  data: x input; y output
function y = fcn(x)
iiuav = 1;
y = x(:,iiuav);

== matlab function run_sim_paper_scenario/choose ksi_est_err 55 ==
  data: x input; y output
function y = fcn(x)
iiuav = 2;
y = x(:,iiuav);

== matlab function run_sim_paper_scenario/choose ksi_est_err 56 ==
  data: x input; y output
function y = fcn(x)
iiuav = 3;
y = x(:,iiuav);

== matlab function run_sim_paper_scenario/choose ksi_est_err 57 ==
  data: x input; y output
function y = fcn(x)
iiuav = 4;
y = x(:,iiuav);

== matlab function run_sim_paper_scenario/choose ksi_est_err 58 ==
  data: x input; y output
function y = fcn(x)
iiuav = 5;
y = x(:,iiuav);

== matlab function run_sim_paper_scenario/cal theta_err_ksi agent 5 ==
  data: alfa_theta input; err_ksi_squ_1_node_5 input; theta_err_ksi_1_5 output; err_ksi_squ_2_node_5 input; err_ksi_vec input; theta_err_ksi_2_5 output
function [theta_err_ksi_1_5, theta_err_ksi_2_5] = fcn(alfa_theta, err_ksi_squ_1_node_5, err_ksi_squ_2_node_5, err_ksi_vec)
iiuav = 5;
theta_err_ksi_1_5 = err_ksi_squ_1_node_5(:) .* ( -1 + 2 ./ ( 1 + exp( -alfa_theta .* err_ksi_vec(:,iiuav) ) ) );
theta_err_ksi_2_5 = err_ksi_squ_2_node_5(:) .* ( -1 + 2 ./ ( 1 + exp( -alfa_theta .* err_ksi_vec(:,iiuav) ) ) );

== matlab function run_sim_paper_scenario/choose ksi_est_err 59 ==
  data: x input; y output
function y = fcn(x)
iiuav = 1;
y = x(:,iiuav);

== matlab function run_sim_paper_scenario/choose ksi_est_err 60 ==
  data: x input; y output
function y = fcn(x)
iiuav = 1;
y = x(:,iiuav);

== matlab function run_sim_paper_scenario/choose ksi_est_err 61 ==
  data: x input; y output
function y = fcn(x)
iiuav = 2;
y = x(:,iiuav);

== matlab function run_sim_paper_scenario/choose ksi_est_err 62 ==
  data: x input; y output
function y = fcn(x)
iiuav = 2;
y = x(:,iiuav);

== matlab function run_sim_paper_scenario/choose ksi_est_err 63 ==
  data: x input; y output
function y = fcn(x)
iiuav = 2;
y = x(:,iiuav);

== matlab function run_sim_paper_scenario/choose ksi_est_err 64 ==
  data: x input; y output
function y = fcn(x)
iiuav = 3;
y = x(:,iiuav);

== matlab function run_sim_paper_scenario/choose ksi_est_err 65 ==
  data: x input; y output
function y = fcn(x)
iiuav = 3;
y = x(:,iiuav);

== matlab function run_sim_paper_scenario/choose ksi_est_err 66 ==
  data: x input; y output
function y = fcn(x)
iiuav = 4;
y = x(:,iiuav);

== matlab function run_sim_paper_scenario/choose ksi_est_err 67 ==
  data: x input; y output
function y = fcn(x)
iiuav = 4;
y = x(:,iiuav);

== matlab function run_sim_paper_scenario/choose ksi_est_err 68 ==
  data: x input; y output
function y = fcn(x)
iiuav = 5;
y = x(:,iiuav);

== matlab function run_sim_paper_scenario/choose ksi_est_err 69 ==
  data: x input; y output
function y = fcn(x)
iiuav = 5;
y = x(:,iiuav);

== matlab function run_sim_paper_scenario/choose ksi_est_err 70 ==
  data: x input; y output
function y = fcn(x)
iiuav = 2;
y = x(:,iiuav);

== matlab function run_sim_paper_scenario/choose ksi_est_err 71 ==
  data: x input; y output
function y = fcn(x)
iiuav = 3;
y = x(:,iiuav);

== matlab function run_sim_paper_scenario/choose ksi_est_err 72 ==
  data: x input; y output
function y = fcn(x)
iiuav = 3;
y = x(:,iiuav);

== matlab function run_sim_paper_scenario/choose ksi_est_err 73 ==
  data: x input; y output
function y = fcn(x)
iiuav = 4;
y = x(:,iiuav);

== matlab function run_sim_paper_scenario/choose ksi_est_err 10 ==
  data: x input; y output
function y = fcn(x)
iiuav = 5;
y = x(:,iiuav);

== matlab function run_sim_paper_scenario/choose ksi_est_err 74 ==
  data: x input; y output
function y = fcn(x)
iiuav = 4;
y = x(:,iiuav);

== matlab function run_sim_paper_scenario/choose ksi_est_err 75 ==
  data: x input; y output
function y = fcn(x)
iiuav = 5;
y = x(:,iiuav);

== matlab function run_sim_paper_scenario/choose ui agent 1 ==
  data: x input; y output
function y = fcn(x)
iiuav = 1;
y = x(:,iiuav);

== matlab function run_sim_paper_scenario/choose ui agent 2 ==
  data: x input; y output
function y = fcn(x)
iiuav = 2;
y = x(:,iiuav);

== matlab function run_sim_paper_scenario/choose ui agent 3 ==
  data: x input; y output
function y = fcn(x)
iiuav = 3;
y = x(:,iiuav);

== matlab function run_sim_paper_scenario/choose ui agent 4 ==
  data: x input; y output
function y = fcn(x)
iiuav = 4;
y = x(:,iiuav);

== matlab function run_sim_paper_scenario/choose ui agent 5 ==
  data: x input; y output
function y = fcn(x)
iiuav = 5;
y = x(:,iiuav);

== matlab function run_sim_paper_scenario/combine Fi_S ==
  data: Fi_S_1 input; Fi_S_2 input; Fi_S_3 input; Fi_S_4 input; Fi_S_5 input; Fi_S_vec output
function Fi_S_vec  = fcn(Fi_S_1, Fi_S_2, Fi_S_3, Fi_S_4, Fi_S_5)
Fi_S_vec = zeros(3,5);
Fi_S_vec(:,1) = Fi_S_1(:);
Fi_S_vec(:,2) = Fi_S_2(:);
Fi_S_vec(:,3) = Fi_S_3(:);
Fi_S_vec(:,4) = Fi_S_4(:);
Fi_S_vec(:,5) = Fi_S_5(:);

== matlab function run_sim_paper_scenario/combine Phi_bar_psi_e ==
  data: Phi_bar_psi_e_node_1 input; Phi_bar_psi_e_node_2 input; Phi_bar_psi_e_node_3 input; Phi_bar_psi_e_node_4 input; Phi_bar_psi_e_node_5 input; Phi_bar_psi_e_vec output
function Phi_bar_psi_e_vec  = fcn(Phi_bar_psi_e_node_1, Phi_bar_psi_e_node_2, Phi_bar_psi_e_node_3, ...
                                                                Phi_bar_psi_e_node_4, Phi_bar_psi_e_node_5)
Phi_bar_psi_e_vec = zeros(3,5);
Phi_bar_psi_e_vec(:,1) = Phi_bar_psi_e_node_1(:);
Phi_bar_psi_e_vec(:,2) = Phi_bar_psi_e_node_2(:);
Phi_bar_psi_e_vec(:,3) = Phi_bar_psi_e_node_3(:);
Phi_bar_psi_e_vec(:,4) = Phi_bar_psi_e_node_4(:);
Phi_bar_psi_e_vec(:,5) = Phi_bar_psi_e_node_5(:);

== matlab function run_sim_paper_scenario/choose ksi_est_err 9 ==
  data: x input; y output
function y = fcn(x)
iiuav = 5;
y = x(:,iiuav);

== matlab function run_sim_paper_scenario/combine Phi_psi_e ==
  data: Phi_psi_e_node_1 input; Phi_psi_e_node_2 input; Phi_psi_e_node_3 input; Phi_psi_e_node_4 input; Phi_psi_e_node_5 input; Phi_psi_e_vec output
function Phi_psi_e_vec  = fcn(Phi_psi_e_node_1, Phi_psi_e_node_2, Phi_psi_e_node_3, ...
                                                        Phi_psi_e_node_4, Phi_psi_e_node_5)
Phi_psi_e_vec = zeros(3,5);
Phi_psi_e_vec(:,1) = Phi_psi_e_node_1(:);
Phi_psi_e_vec(:,2) = Phi_psi_e_node_2(:);
Phi_psi_e_vec(:,3) = Phi_psi_e_node_3(:);
Phi_psi_e_vec(:,4) = Phi_psi_e_node_4(:);
Phi_psi_e_vec(:,5) = Phi_psi_e_node_5(:);

== matlab function run_sim_paper_scenario/combine Qci Rci ==
  data: Qci_1 input; Qci_vec output; Qci_2 input; Qci_3 input; Qci_4 input; Qci_5 input; Rci_1 input; Rci_2 input; Rci_3 input; Rci_4 input; Rci_5 input; Rci_vec output
function [Qci_vec, Rci_vec] = fcn(Qci_1, Qci_2, Qci_3, Qci_4, Qci_5, ...
                                                            Rci_1, Rci_2, Rci_3, Rci_4, Rci_5)

Qci_vec = zeros(4,5);
Qci_vec(:,1) = Qci_1(:);
Qci_vec(:,2) = Qci_2(:);
Qci_vec(:,3) = Qci_3(:);
Qci_vec(:,4) = Qci_4(:);
Qci_vec(:,5) = Qci_5(:);

Rci_vec = zeros(3,3,5);
Rci_vec(:,:,1) = Rci_1;
Rci_vec(:,:,2) = Rci_2;
Rci_vec(:,:,3) = Rci_3;
Rci_vec(:,:,4) = Rci_4;
Rci_vec(:,:,5) = Rci_5;

== matlab function run_sim_paper_scenario/combine Qci Rci1 ==
  data: V_Phi_Rei_1 input; V_Phi_Rei_vec output; V_Phi_Rei_2 input; V_Phi_Rei_3 input; V_Phi_Rei_4 input; V_Phi_Rei_5 input
function V_Phi_Rei_vec = fcn(V_Phi_Rei_1, V_Phi_Rei_2, V_Phi_Rei_3, V_Phi_Rei_4, V_Phi_Rei_5)
V_Phi_Rei_vec = [V_Phi_Rei_1(:), V_Phi_Rei_2(:), V_Phi_Rei_3(:), V_Phi_Rei_4(:), V_Phi_Rei_5(:)];

== matlab function run_sim_paper_scenario/combine Qi Ri ==
  data: Qi_1 input; Qi_vec output; Qi_2 input; Qi_3 input; Qi_4 input; Qi_5 input; Ri_1 input; Ri_2 input; Ri_3 input; Ri_4 input; Ri_5 input; Ri_vec output
function [Qi_vec, Ri_vec] = fcn(Qi_1, Qi_2, Qi_3, Qi_4, Qi_5, ...
                                                        Ri_1, Ri_2, Ri_3, Ri_4, Ri_5)

Qi_vec = zeros(4,5);
Qi_vec(:,1) = Qi_1(:);
Qi_vec(:,2) = Qi_2(:);
Qi_vec(:,3) = Qi_3(:);
Qi_vec(:,4) = Qi_4(:);
Qi_vec(:,5) = Qi_5(:);

Ri_vec = zeros(3,3,5);
Ri_vec(:,:,1) = Ri_1;
Ri_vec(:,:,2) = Ri_2;
Ri_vec(:,:,3) = Ri_3;
Ri_vec(:,:,4) = Ri_4;
Ri_vec(:,:,5) = Ri_5;

== matlab function run_sim_paper_scenario/combine S_bar ==
  data: S_bar_node_1 input; S_bar_node_2 input; S_bar_node_3 input; S_bar_node_4 input; S_bar_node_5 input; S_bar_vec output
function S_bar_vec  = fcn(S_bar_node_1, S_bar_node_2, S_bar_node_3, ...
                                                S_bar_node_4, S_bar_node_5)
S_bar_vec = zeros(3,5);
S_bar_vec(:,1) = S_bar_node_1(:);
S_bar_vec(:,2) = S_bar_node_2(:);
S_bar_vec(:,3) = S_bar_node_3(:);
S_bar_vec(:,4) = S_bar_node_4(:);
S_bar_vec(:,5) = S_bar_node_5(:);

== matlab function run_sim_paper_scenario/combine Si ==
  data: Si_1 input; Si_2 input; Si_3 input; Si_4 input; Si_5 input; Si_vec output
function Si_vec  = fcn(Si_1, Si_2, Si_3, Si_4, Si_5)
Si_vec = zeros(3,5);
Si_vec(:,1) = Si_1(:);
Si_vec(:,2) = Si_2(:);
Si_vec(:,3) = Si_3(:);
Si_vec(:,4) = Si_4(:);
Si_vec(:,5) = Si_5(:);

== matlab function run_sim_paper_scenario/trans to column8 ==
  data: x input; y output
function y = fcn(x)
y = x(:);

== matlab function run_sim_paper_scenario/combine Si_squ_beta_w_1 ==
  data: Si_squ_beta_w_1_node_1 input; Si_squ_beta_w_1_node_2 input; Si_squ_beta_w_1_node_3 input; Si_squ_beta_w_1_node_4 input; Si_squ_beta_w_1_node_5 input; Si_squ_beta_w_1_vec output
function Si_squ_beta_w_1_vec  = fcn(Si_squ_beta_w_1_node_1, Si_squ_beta_w_1_node_2, Si_squ_beta_w_1_node_3, ...
                                                                    Si_squ_beta_w_1_node_4, Si_squ_beta_w_1_node_5)
Si_squ_beta_w_1_vec = zeros(3,5);
Si_squ_beta_w_1_vec(:,1) = Si_squ_beta_w_1_node_1(:);
Si_squ_beta_w_1_vec(:,2) = Si_squ_beta_w_1_node_2(:);
Si_squ_beta_w_1_vec(:,3) = Si_squ_beta_w_1_node_3(:);
Si_squ_beta_w_1_vec(:,4) = Si_squ_beta_w_1_node_4(:);
Si_squ_beta_w_1_vec(:,5) = Si_squ_beta_w_1_node_5(:);

== matlab function run_sim_paper_scenario/combine Si_squ_beta_w_2 ==
  data: Si_squ_beta_w_2_node_1 input; Si_squ_beta_w_2_node_2 input; Si_squ_beta_w_2_node_3 input; Si_squ_beta_w_2_node_4 input; Si_squ_beta_w_2_node_5 input; Si_squ_beta_w_2_vec output
function Si_squ_beta_w_2_vec  = fcn(Si_squ_beta_w_2_node_1, Si_squ_beta_w_2_node_2, Si_squ_beta_w_2_node_3, ...
                                                                    Si_squ_beta_w_2_node_4, Si_squ_beta_w_2_node_5)
Si_squ_beta_w_2_vec = zeros(3,5);
Si_squ_beta_w_2_vec(:,1) = Si_squ_beta_w_2_node_1(:);
Si_squ_beta_w_2_vec(:,2) = Si_squ_beta_w_2_node_2(:);
Si_squ_beta_w_2_vec(:,3) = Si_squ_beta_w_2_node_3(:);
Si_squ_beta_w_2_vec(:,4) = Si_squ_beta_w_2_node_4(:);
Si_squ_beta_w_2_vec(:,5) = Si_squ_beta_w_2_node_5(:);

== matlab function run_sim_paper_scenario/combine V_Phi_Rei_squ_2p ==
  data: V_Phi_Rei_squ_2p_node_1 input; V_Phi_Rei_squ_2p_node_2 input; V_Phi_Rei_squ_2p_node_3 input; V_Phi_Rei_squ_2p_node_4 input; V_Phi_Rei_squ_2p_node_5 input; V_Phi_Rei_squ_2p_vec output
function V_Phi_Rei_squ_2p_vec  = fcn(V_Phi_Rei_squ_2p_node_1, V_Phi_Rei_squ_2p_node_2, V_Phi_Rei_squ_2p_node_3, ...
                                                                        V_Phi_Rei_squ_2p_node_4, V_Phi_Rei_squ_2p_node_5)
V_Phi_Rei_squ_2p_vec = zeros(3,5);
V_Phi_Rei_squ_2p_vec(:,1) = V_Phi_Rei_squ_2p_node_1(:);
V_Phi_Rei_squ_2p_vec(:,2) = V_Phi_Rei_squ_2p_node_2(:);
V_Phi_Rei_squ_2p_vec(:,3) = V_Phi_Rei_squ_2p_node_3(:);
V_Phi_Rei_squ_2p_vec(:,4) = V_Phi_Rei_squ_2p_node_4(:);
V_Phi_Rei_squ_2p_vec(:,5) = V_Phi_Rei_squ_2p_node_5(:);

== matlab function run_sim_paper_scenario/combine V_Phi_Rei_squ_p_min_1 ==
  data: V_Phi_Rei_squ_p_min_1_node_1 input; V_Phi_Rei_squ_p_min_1_node_2 input; V_Phi_Rei_squ_p_min_1_node_3 input; V_Phi_Rei_squ_p_min_1_node_4 input; V_Phi_Rei_squ_p_min_1_node_5 input; V_Phi_Rei_squ_p_min_1_vec output
function V_Phi_Rei_squ_p_min_1_vec  = fcn(V_Phi_Rei_squ_p_min_1_node_1, V_Phi_Rei_squ_p_min_1_node_2, V_Phi_Rei_squ_p_min_1_node_3, ...
                                                                                V_Phi_Rei_squ_p_min_1_node_4, V_Phi_Rei_squ_p_min_1_node_5)
V_Phi_Rei_squ_p_min_1_vec = zeros(3,5);
V_Phi_Rei_squ_p_min_1_vec(:,1) = V_Phi_Rei_squ_p_min_1_node_1(:);
V_Phi_Rei_squ_p_min_1_vec(:,2) = V_Phi_Rei_squ_p_min_1_node_2(:);
V_Phi_Rei_squ_p_min_1_vec(:,3) = V_Phi_Rei_squ_p_min_1_node_3(:);
V_Phi_Rei_squ_p_min_1_vec(:,4) = V_Phi_Rei_squ_p_min_1_node_4(:);
V_Phi_Rei_squ_p_min_1_vec(:,5) = V_Phi_Rei_squ_p_min_1_node_5(:);

== matlab function run_sim_paper_scenario/combine V_Phi_Rei_squ_p_plus_1 ==
  data: V_Phi_Rei_squ_p_plus_1_node_1 input; V_Phi_Rei_squ_p_plus_1_node_2 input; V_Phi_Rei_squ_p_plus_1_node_3 input; V_Phi_Rei_squ_p_plus_1_node_4 input; V_Phi_Rei_squ_p_plus_1_node_5 input; V_Phi_Rei_squ_p_plus_1_vec output
function V_Phi_Rei_squ_p_plus_1_vec  = fcn(V_Phi_Rei_squ_p_plus_1_node_1, V_Phi_Rei_squ_p_plus_1_node_2, V_Phi_Rei_squ_p_plus_1_node_3, ...
                                                                                V_Phi_Rei_squ_p_plus_1_node_4, V_Phi_Rei_squ_p_plus_1_node_5)
V_Phi_Rei_squ_p_plus_1_vec = zeros(3,5);
V_Phi_Rei_squ_p_plus_1_vec(:,1) = V_Phi_Rei_squ_p_plus_1_node_1(:);
V_Phi_Rei_squ_p_plus_1_vec(:,2) = V_Phi_Rei_squ_p_plus_1_node_2(:);
V_Phi_Rei_squ_p_plus_1_vec(:,3) = V_Phi_Rei_squ_p_plus_1_node_3(:);
V_Phi_Rei_squ_p_plus_1_vec(:,4) = V_Phi_Rei_squ_p_plus_1_node_4(:);
V_Phi_Rei_squ_p_plus_1_vec(:,5) = V_Phi_Rei_squ_p_plus_1_node_5(:);
